simulink model "Kontrollu_Boost_Converter"  (R2022a)
settings: Solver=VariableStepAuto  StartTime=0.0  StopTime=3.0  RelTol=1e-3
libraries: spsSeriesRLCBranchLib x6, spsBreakerLib x3, spsCurrentMeasurementLib x1, spsDCVoltageSourceLib x1, spsDiodeLib x1, spsMosfetLib x1, spsVoltageMeasurementLib x1, spspowerguiLib x1, spsTriangleGeneratorLib x1
settings Model: Creator=unaly  LastModifiedBy=unaly

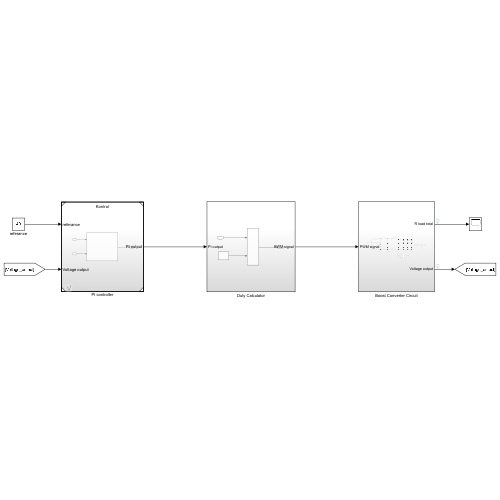
[thumbnail: Simulink's stored preview of the top-level diagram]
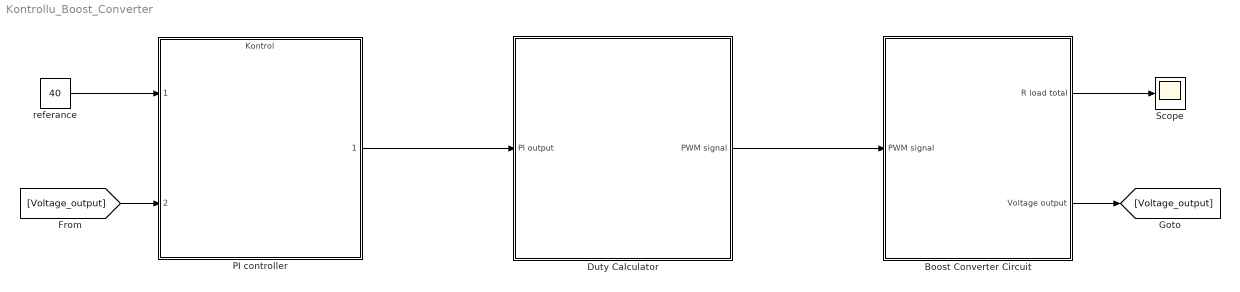
== system Kontrollu_Boost_Converter ==
  Boost Converter Circuit : Subsystem
  Duty Calculator : Subsystem
  PI controller : ModelReference  ModelNameDialog=Kontrol.slx  SimulationMode=Normal  ModelReferenceVersion=1.4
  Scope : Scope
  referance : Constant  Value=40
  wires:
  Duty Calculator/1(PWM signal) -> Boost Converter Circuit/1(PWM signal)
  PI controller/1 -> Duty Calculator/1(PI output)
  Boost Converter Circuit/2(Voltage output) -> [Voltage_output]
  [Voltage_output] -> PI controller/2
  referance/1 -> PI controller/1
  Boost Converter Circuit/1(R load total) -> Scope/1

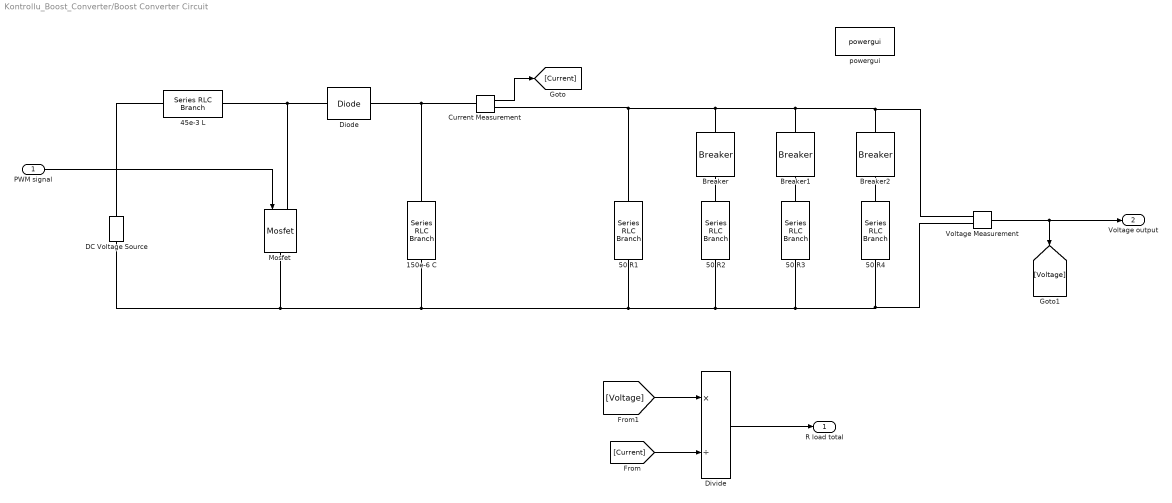
== system Kontrollu_Boost_Converter/Boost Converter Circuit ==
  PWM signal : Inport
  150e-6 C : spsSeriesRLCBranchLib/Series RLC Branch  LConnTagsString=__new0  RConnTagsString=__new0  BranchType=C  Resistance=1  Inductance=1e-3  SetiL0=off  InitialCurrent=0  Capacitance=150e-6  Setx0=off  InitialVoltage=0  Measurements=None
  45e-3 L : spsSeriesRLCBranchLib/Series RLC Branch  LConnTagsString=__new0  RConnTagsString=__new0  BranchType=L  Resistance=1  Inductance=45e-3  SetiL0=off  InitialCurrent=0  Capacitance=1e-6  Setx0=off  InitialVoltage=0  Measurements=None
  50 R{1..4} (4 alike) : spsSeriesRLCBranchLib/Series RLC Branch  LConnTagsString=__new0  RConnTagsString=__new0  BranchType=R  Resistance=50  Inductance=1e-3  SetiL0=off  InitialCurrent=0  Capacitance=1e-6  Setx0=off  InitialVoltage=0  Measurements=None
  Breaker : spsBreakerLib/Breaker  InitialState=0  SwitchingTimes="[0.5  4]"  External=off  BreakerResistance=0.01  SnubberResistance=1e6  SnubberCapacitance=inf  Measurements=None  MoreParameters=on  NoBreakLoop=off
      settings: SourceProductBaseCode=PS
  Breaker1 : spsBreakerLib/Breaker  InitialState=0  SwitchingTimes="[1  4]"  External=off  BreakerResistance=0.01  SnubberResistance=1e6  SnubberCapacitance=inf  Measurements=None  MoreParameters=on  NoBreakLoop=off
      settings: SourceProductBaseCode=PS
  Breaker2 : spsBreakerLib/Breaker  InitialState=0  SwitchingTimes="[2  4]"  External=off  BreakerResistance=0.01  SnubberResistance=1e6  SnubberCapacitance=inf  Measurements=None  MoreParameters=on  NoBreakLoop=off
      settings: SourceProductBaseCode=PS
  Current Measurement : spsCurrentMeasurementLib/Current Measurement  PhasorSimulation=off  OutputType=Complex  PSBequivalent=0
  DC Voltage Source : spsDCVoltageSourceLib/DC Voltage Source  Amplitude=15  Measurements=None
  Diode : spsDiodeLib/Diode  Ron=0.001  Lon=0  Vf=0.8  IC=0  UseSnubber=0  Rs=500  Cs=250e-9  Measurements=off
  Divide : Product  Inputs=*/
  Mosfet : spsMosfetLib/Mosfet  Ron=0.1  Lon=0  Rd=0.01  Vfd=0  IC=0  Rs=1e5  Cs=inf  Measurements=off
  Voltage Measurement : spsVoltageMeasurementLib/Voltage Measurement  PhasorSimulation=off  OutputType=Complex  PSBequivalent=0
  powergui : spspowerguiLib/powergui  Priority=1  SimulationMode=Continuous  SampleTime=50e-6  frequency=60  Iterations=50  frequencyindice=0  Pbase=100e6  ErrMax=1e-4  UnitsV=kV  UnitsW=MW  buscounter=0  FunctionMessages=off  echomessages=off  EnableUseOfTLC=off  CurrentSourceSwitches=off  DisableSnubberDevices=off  DisableRonSwitches=off  DisableVfSwitches=off  DisplayEquations=off  AutomaticDiscreteSolvers=off  SolverType=Tustin/Backward Euler (TBE)  Interpol=off  ExternalGateDelay=off  methode=off  Ts=100  x0status=blocks  SPID=on  SwTol=0  HookPort=off  NonlinearTolerance=1e-4  nMaxIteration=100  ContinueOnMaxIteration=off  RestoreLinks=warning  ResistiveCurrentMeasurement=off  Frange=[0:2:500]  Ylog=off  Xlog=on  ShowGrid=off  save=off  variable=ZData  structure=0  ZoomFFT=off  StartTime=0.0  cycles=1  DisplayStyle=1  fundamental=60  FreqAxis=off  MaxFrequency=1000  frequencyindicesteady=1  RmsSteady=1  display=off
  R load total : Outport
  Voltage output : Outport  Port=2
  wires:
  [Current] -> Divide/2
  [Voltage] -> Divide/1
  Voltage Measurement/1 -> Voltage output/1, [Voltage]
  Divide/1 -> R load total/1
  Current Measurement/1 -> [Current]
  PWM signal/1 -> Mosfet/1
  connections:
  Current Measurement/RConn1 -- Voltage Measurement/LConn1 -- Breaker2/LConn1 -- Breaker1/LConn1 -- Breaker/LConn1 -- 50 R1/LConn1
  50 R4/LConn1 -- Breaker2/RConn1
  Diode/RConn1 -- Current Measurement/LConn1 -- 150e-6 C/LConn1
  50 R2/LConn1 -- Breaker/RConn1
  DC Voltage Source/LConn1 -- Mosfet/RConn1 -- Voltage Measurement/LConn2 -- 50 R4/RConn1 -- 50 R3/RConn1 -- 50 R2/RConn1 -- 50 R1/RConn1 -- 150e-6 C/RConn1
  50 R3/LConn1 -- Breaker1/RConn1
  DC Voltage Source/RConn1 -- 45e-3 L/LConn1
  45e-3 L/RConn1 -- Diode/LConn1 -- Mosfet/LConn1

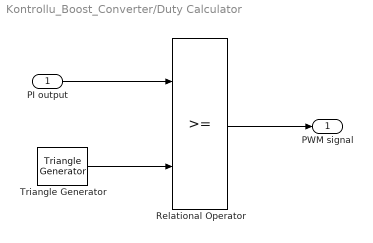
== system Kontrollu_Boost_Converter/Duty Calculator ==
  PI output : Inport
  Relational Operator : RelationalOperator  OutDataTypeStr=boolean  RndMeth=Simplest  InputSameDT=off
  Triangle Generator : spsTriangleGeneratorLib/Triangle Generator  Freq=25e3  Phase=0  Ts=0
  PWM signal : Outport
  wires:
  Relational Operator/1 -> PWM signal/1
  PI output/1 -> Relational Operator/1
  Triangle Generator/1 -> Relational Operator/2
